simulink model "ACCM_SWC"  (R2022b)
settings: configuration reference "ACC_AutosarConfig" (kept outside this file)
model workspace (MATLAB code in the model file):
  | cmdLim = Simulink.Parameter;
  | cmdLim.Value = 15;
  | cmdLim.Description = 'Limit for controlling the maximum surface command angle.';
  | cmdLim.Min = 0;
  | cmdLim.Max = 90;
  | cmdLim.DocUnits = 'deg';
  | 
  | dispGain = Simulink.Parameter;
  | dispGain.Value = 0.75;
  | dispGain.Description = 'Gain applied to the displacement error.';
  | dispGain.Min = 0;
  | dispGain.Max = [];
  | dispGain.DocUnits = 'deg/sec/deg';
  | 
  | dispLim = Simulink.Parameter;
  | dispLim.Value = 30;
  | dispLim.Description = 'Limit for controlling the maximum commanded angle.';
  | dispLim.Min = 0;
  | dispLim.Max = 180;
  | dispLim.DocUnits = 'deg';
  | 
  | intGain = Simulink.Parameter;
  | intGain.Value = 0.5;
  | intGain.Description = 'Gain applied to the integral error.';
  | intGain.Min = 0;
  | intGain.Max = [];
  | intGain.DocUnits = 'deg/sec/deg/sec';
  | 
  | intLim = Simulink.Parameter;
  | intLim.Value = 5;
  | intLim.Description = 'Limit for controlling the maximum commanded angle.';
  | intLim.Min = 0;
  | intLim.Max = 90;
  | intLim.DocUnits = 'deg';
  | 
  | rateGain = Simulink.Parameter;
  | rateGain.Value = 2;
  | rateGain.Description = 'Gain applied to the rate error.';
  | rateGain.Min = 0;
  | rateGain.Max = [];
  | rateGain.DocUnits = 'deg/deg/sec';
  | 
  | rateLim = Simulink.Parameter;
  | rateLim.Value = 6;
  | rateLim.Description = 'Limit for controlling the maximum commanded angle.';
  | rateLim.Min = 0;
  | rateLim.Max = 180;
  | rateLim.DocUnits = 'deg/sec';
  | 
  | hdgGain = Simulink.Parameter;
  | hdgGain.Value = 0.015;
values from neighbouring files (symbols this model uses):
  ACC_SampleTime = 0.01    [ACC_DD.sldd]
undefined symbols (not defined in the file or in its folder): ACC_Mode
libraries: autosarlibdem x1
settings Model: RequirementInfo={} %GIDa_fe9045fd_0412_4b6e_8206_617cc20e6fde  DataDictionary=ACC_DD.sldd  FPTRunName=Active  Creator=MAAM  LastModifiedBy=MAAM
settings ConfigSetRef: SourceName=ACC_AutosarConfig

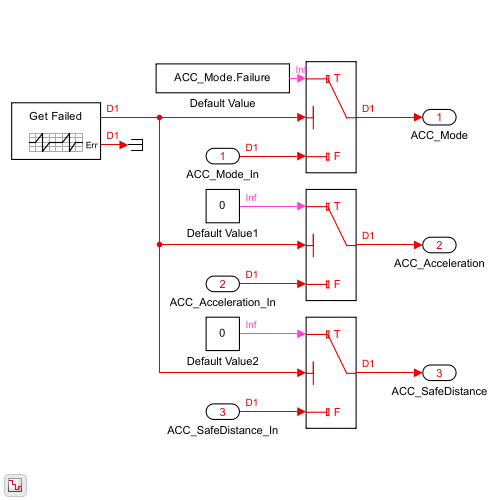
[thumbnail: Simulink's stored preview of the top-level diagram]
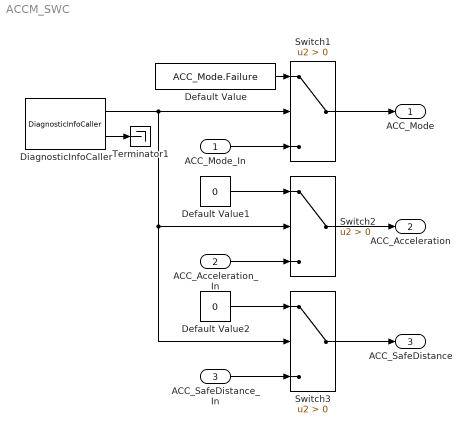
== system ACCM_SWC ==
  ACC_Mode_In : Inport
  ACC_Acceleration_In : Inport  Port=2  OutDataTypeStr=single  SampleTime=ACC_SampleTime
  ACC_SafeDistance_In : Inport  Port=3  OutDataTypeStr=single  SampleTime=ACC_SampleTime
  Default Value : Constant  Value=ACC_Mode.Failure
  Default Value1 : Constant  Value=0  OutDataTypeStr=single
  Default Value2 : Constant  Value=0  OutDataTypeStr=single
  DiagnosticInfoCaller : autosarlibdem/DiagnosticInfoCaller  PortName=ACC_Fail  Operation=GetEventFailed  st=-1  ServiceImpl=autosar.bsw.DemDiagnosticInfo
  Switch1 : Switch  Criteria=u2 > Threshold  SaturateOnIntegerOverflow=off  InputSameDT=off
  Switch2 : Switch  Criteria=u2 > Threshold  SaturateOnIntegerOverflow=off  InputSameDT=off
  Switch3 : Switch  Criteria=u2 > Threshold  SaturateOnIntegerOverflow=off  InputSameDT=off
  Terminator1 : Terminator
  ACC_Mode : Outport
  ACC_Acceleration : Outport  Port=2
  ACC_SafeDistance : Outport  Port=3
  wires:
  DiagnosticInfoCaller/2 -> Terminator1/1
  Default Value/1 -> Switch1/1
  Switch1/1 -> ACC_Mode/1
  ACC_Mode_In/1 -> Switch1/3
  ACC_Acceleration_In/1 -> Switch2/3
  Switch2/1 -> ACC_Acceleration/1
  Default Value1/1 -> Switch2/1
  DiagnosticInfoCaller/1 -> Switch3/2, Switch2/2, Switch1/2
  Default Value2/1 -> Switch3/1
  Switch3/1 -> ACC_SafeDistance/1
  ACC_SafeDistance_In/1 -> Switch3/3
